simulink model "My_Model"  (R2022a)
settings: Solver=VariableStepAuto  StartTime=0.0  StopTime=10.0  RelTol=1e-3
libraries: neural x1294, spsSeriesRLCBranchLib x16, spsDiodeLib x14, spsMosfetLib x9, spsVoltageMeasurementLib x9, powerlib_extras x8, spsThreePhaseVIMeasurementLib x7, spsCurrentMeasurementLib x4, spsPVArrayLib x4, spsPWMGeneratorDCDCLib x4, spsTHDLib x4, spsThreePhaseParallelRLCBranchLib x3
(part 1 of 41)
settings Model: Creator=Irfan  LastModifiedBy=Irfan
settings SolverCC: MaxZcPerStep=1

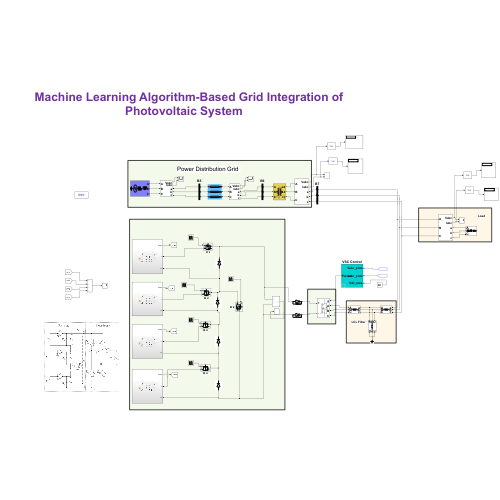
[thumbnail: Simulink's stored preview of the top-level diagram]
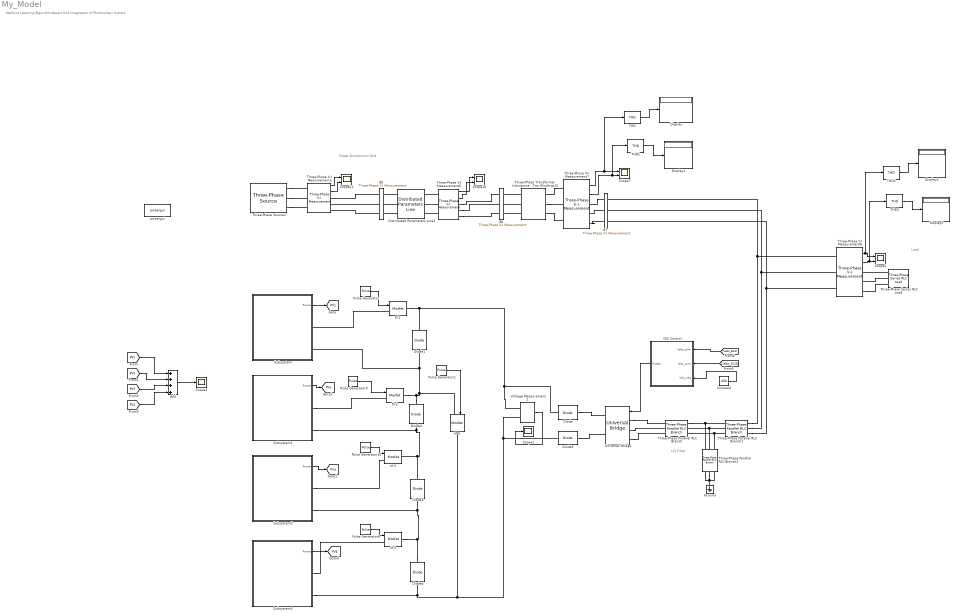
== system My_Model ==
  note: Load
  note: LCL Filter
  note: Machine Learning Algorithm-Based Grid Integration of Photovoltaic System
  note: Power Distribution Grid
  Add : Sum  Inputs=++++
  B5 : spsThreePhaseVIMeasurementLib/Three-Phase V-I Measurement  VoltageMeasurement=no  SetLabelV=off  LabelV=Vabc_B12  Vpu=off  VpuLL=off  CurrentMeasurement=no  SetLabelI=off  LabelI=A1  Ipu=off  Pbase=100e6  Vbase=25e3  OutputType=Magnitude  PhasorSimulation=off  PSBequivalent=0
  B6 : spsThreePhaseVIMeasurementLib/Three-Phase V-I Measurement  VoltageMeasurement=no  SetLabelV=off  LabelV=Vabc_B12  Vpu=off  VpuLL=off  CurrentMeasurement=no  SetLabelI=off  LabelI=A1  Ipu=off  Pbase=100e6  Vbase=440  OutputType=Magnitude  PhasorSimulation=off  PSBequivalent=0
  B7 : spsThreePhaseVIMeasurementLib/Three-Phase V-I Measurement  VoltageMeasurement=phase-to-ground  SetLabelV=on  LabelV=Vabc_B13  Vpu=off  VpuLL=off  CurrentMeasurement=yes  SetLabelI=on  LabelI=Iabc_b13  Ipu=off  Pbase=100e6  Vbase=440  OutputType=Magnitude  PhasorSimulation=off  PSBequivalent=0
  Constant : Constant  Value=400
  Diode : spsDiodeLib/Diode  Ron=0.001  Lon=0  Vf=0.8  IC=0  UseSnubber=0  Rs=500  Cs=250e-9  Measurements=off
  Diode{1..4} (4 alike) : spsDiodeLib/Diode  Ron=0.001  Lon=0  Vf=0.7  IC=0  UseSnubber=0  Rs=500  Cs=0  Measurements=off
  Diode5 : spsDiodeLib/Diode  Ron=0.001  Lon=0  Vf=0.8  IC=0  UseSnubber=0  Rs=500  Cs=250e-9  Measurements=off
  Display{,1..3} (4 alike) : Display
  Distributed Parameters Line1 : spsDistributedParametersLineLib/Distributed Parameters Line  Phases=3  Length=100  Frequency=50  Resistance=[0.01273 0.3864]  Inductance="[0.9337e-3  4.1264e-3]"  Capacitance=[12.74e-9 7.751e-9]  x1=[-0.0006 -0.058188576465129 21083.6440305902 -61014.2835927059;-0.00055 -0.0555200850052596 22039.4110790569 -60675.591993026;-0.0005 -0.0528378947951801 22989.7402326226 -60321.9295989302;-0.00045 -0.0501426676251903 23934.3970117888 -59953.3836713222;-0.0004 -0.0474350685022648 24873.1483366304 -59570.0451433951;-0.00035 -0.0447157654859725 25805.7625843049 -59172.0085981946;-0.0003 -0.0419854295236429 26732.0096462016 -58759.3722452823;-0.00025 -0.0392447342848198 27651.6609847177 -58332.2378965037;-0.0002 -0.0364943559950435 28564.4896896465 -57890.7109408683;-0.00015 -0.0337349732690022 29470.2705341641 -57434.9003185455;-0.0001 -0.0309672669430941 30368.7800304004 -56964.9184939859;-5e-05 -0.0281919199074408 31259.7964845821 -56480.8814281723]  x2=[-0.0006 -0.327906164256312 21190.0392255692 -61379.0148200665;-0.00055 -0.31698546988336 22151.5200142409 -61038.6090322539;-0.0005 -0.305986564088869 23107.5352468095 -60683.1428810029;-0.00045 -0.294912160688264 24057.8490408213 -60312.7040722674;-0.0004 -0.283764992124876 25002.2269205677 -59927.3840062804;-0.00035 -0.272547808795747 25940.4358749378 -59527.2777550025;-0.0003 -0.261263378373018 26872.2444149108 -59112.4840386644;-0.00025 -0.249914485121043 27797.4226306725 -58683.1052014089;-0.0002 -0.238503929209416 28715.7422483418 -58239.247186039;-0.00015 -0.227034526022067 29626.9766862941 -57781.0195078786;-0.0001 -0.215509105462612 30530.9011110672 -57308.5352277505;-5e-05 -0.203930511256117 31427.2924928347 -56821.910924081]  x3=[-0.0006 -0.00428228203564021 53.1676137199478 -232.949570816253;-0.00055 -0.0042908783266208 56.8201229832142 -232.085797433882;-0.0005 -0.00429841590758009 60.4586127313522 -231.164760353768;-0.00045 -0.00430489291873276 64.0821852214604 -230.186686828029;-0.0004 -0.00431030776197323 67.6899463912475 -229.151818181673;-0.00035 -0.00431465910126995 71.2810060796291 -228.060409753053;-0.0003 -0.00431794586299507 74.854478246361 -226.912730830867;-0.00025 -0.0043201672361893 78.4094811906572 -225.709064587717;-0.0002 -0.00432132267276205 81.9451377687359 -224.449708010237;-0.00015 -0.00432141188762664 85.4605756102416 -223.134971825819;-0.0001 -0.00432043485877063 88.9549273334895 -221.765180425943;-5e-05 -0.00431839182726127 92.4273307594791 -220.34067178614]  x4=[-0.0006 0.00367124666063104 77.9758993188108 -226.009964584727;-0.00055 0.00369703359433742 81.5162088738942 -224.757235875746;-0.0005 0.00372190834032431 85.0364055241912 -223.449051681928;-0.00045 0.00374586476112033 88.5356207138521 -222.085734778147;-0.0004 0.00376889694583712 92.0129910638889 -220.66762154245;-0.00035 0.00379099921162774 95.4676585852005 -219.195061873057;-0.0003 0.00381216610508883 98.8987708902695 -217.668419102034;-0.00025 0.00383239240360616 102.305481403475 -216.08806990564;-0.0002 0.00385167311664321 105.686949569975 -214.454404211391;-0.00015 0.00387000348697256 109.042341063096 -212.767825101854;-0.0001 0.0038873789918496 112.370827990194 -211.028748715186;-5e-05 0.0039037953441285 115.671589096928 -209.237604142463]  x5=0.000565541566995743  V1=[0 0 0 3.131e-09 6.455e+04 6.455e+04;0 0 0 314.2 314.2 314.2;1.571 1.571 1.571 -0.216 0.4129 -1.158]  V2=[0 0 0 1.333e-08 6.493e+04 6.493e+04;0 0 0 314.2 314.2 314.2;1.571 1.571 1.571 -0.3355 0.4126 -1.158]  I1=[0 0 0 7.522e-11 238.9 238.9;0 0 0 314.2 314.2 314.2;1.571 1.571 1.571 -1.605 0.3047 -1.266]  I2=[0 0 0 7.015e-11 239.1 239.1;0 0 0 314.2 314.2 314.2;1.571 1.571 1.571 1.244 0.4122 -1.159]  nHarmo=2  Measurements=None  Decoupling=off  VsMag0=0  VrMag0=0  VsAngle0=0  VrAngle0=0  IsMag0=0  IrMag0=0  IsAngle0=0  IrAngle0=0
      settings: SourceProductBaseCode=PS
  Ground : spsGroundLib/Ground  LConnTagsString=a
  M {1..4,9} (5 alike) : spsMosfetLib/Mosfet  Ron=0.1  Lon=0  Rd=0.01  Vfd=0  IC=0  Rs=1e5  Cs=inf  Measurements=off
  Pulse Generator : DiscretePulseGenerator  PulseType=Time based  Period=0.01  PulseWidth=99.999999
  Pulse Generator1 : DiscretePulseGenerator  PulseType=Time based  Amplitude=0  Period=0.01  PulseWidth=50  PhaseDelay=0.0026
  Pulse Generator10 : DiscretePulseGenerator  PulseType=Time based  Period=0.01  PulseWidth=50  PhaseDelay=0.0026
  Pulse Generator8 : DiscretePulseGenerator  PulseType=Time based  Period=0.01  PulseWidth=25  PhaseDelay=0.0039
  Pulse Generator9 : DiscretePulseGenerator  PulseType=Time based  Period=0.01  PulseWidth=75  PhaseDelay=0.0013
  Scope1 : Scope
  Scope{5,7,10..11} (4 alike) : Scope  NumInputPorts=2
  Scope2 : Scope
  Subsystem : Subsystem
  Subsystem1 : Subsystem
  Subsystem2 : Subsystem
  Subsystem3 : Subsystem
  THD{,1..3} (4 alike) : spsTHDLib/THD  Freq=60  Ts=0
      settings: SourceProductBaseCode=PS
  Three-Phase Parallel RLC Branch : spsThreePhaseParallelRLCBranchLib/Three-Phase Parallel RLC Branch  LConnTagsString=A|B|C  RConnTagsString=A|B|C  BranchType=L  Resistance=1  Inductance=2e-1  Capacitance=1e-6  Measurements=None
      settings: SourceProductBaseCode=PS
  Three-Phase Parallel RLC Branch1 : spsThreePhaseParallelRLCBranchLib/Three-Phase Parallel RLC Branch  LConnTagsString=A|B|C  RConnTagsString=A|B|C  BranchType=L  Resistance=1  Inductance=2e-1  Capacitance=1e-6  Measurements=None
      settings: SourceProductBaseCode=PS
  Three-Phase Parallel RLC Branch2 : spsThreePhaseParallelRLCBranchLib/Three-Phase Parallel RLC Branch  LConnTagsString=A|B|C  RConnTagsString=A|B|C  BranchType=C  Resistance=1  Inductance=1e-3  Capacitance=500e-5  Measurements=None
      settings: SourceProductBaseCode=PS
  Three-Phase Series RLC Load : spsThreePhaseSeriesRLCLoadLib/Three-Phase Series RLC Load  LConnTagsString=A|B|C  Configuration=Y (grounded)  NominalVoltage=440  Vabc=[440 440 440]  Vabcp=[1e3 1e3 1e3]  NominalFrequency=50  UnbalancedPower=on  ActivePower=10e3  InductivePower=1000  CapacitivePower=1000  Pabc=[10e3 9e3 11e3]  QLabc=[100 90 110]  QCabc=[100 90 110]  Pabcp=[10e3 9e3 11e3]  QLabcp=[100 90 110]  QCabcp=[100 90 110]  Measurements=None  LoadType=constant Z
  Three-Phase V-I Measurement5 : spsThreePhaseVIMeasurementLib/Three-Phase V-I Measurement  VoltageMeasurement=phase-to-ground  SetLabelV=off  LabelV=Vabc  Vpu=off  VpuLL=off  CurrentMeasurement=yes  SetLabelI=off  LabelI=Iabc  Ipu=off  Pbase=100e6  Vbase=500e3  OutputType=Complex  PhasorSimulation=off  PSBequivalent=0
  Three-Phase V-I Measurement6 : spsThreePhaseVIMeasurementLib/Three-Phase V-I Measurement  VoltageMeasurement=phase-to-ground  SetLabelV=off  LabelV=Vabc  Vpu=off  VpuLL=off  CurrentMeasurement=yes  SetLabelI=off  LabelI=Iabc  Ipu=off  Pbase=100e6  Vbase=500e3  OutputType=Complex  PhasorSimulation=off  PSBequivalent=0
  Three-Phase V-I Measurement7 : spsThreePhaseVIMeasurementLib/Three-Phase V-I Measurement  VoltageMeasurement=phase-to-phase  SetLabelV=off  LabelV=Vabc_b1  Vpu=off  VpuLL=off  CurrentMeasurement=yes  SetLabelI=off  LabelI=Iabc_b1  Ipu=off  Pbase=100e6  Vbase=500e3  OutputType=Complex  PhasorSimulation=off  PSBequivalent=0
  Three-Phase V-I Measurement8 : spsThreePhaseVIMeasurementLib/Three-Phase V-I Measurement  VoltageMeasurement=phase-to-phase  SetLabelV=off  LabelV=Vabc_b1  Vpu=off  VpuLL=off  CurrentMeasurement=yes  SetLabelI=off  LabelI=Iabc_b1  Ipu=off  Pbase=100e6  Vbase=500e3  OutputType=Complex  PhasorSimulation=off  PSBequivalent=0
  Three-Phase Source1 : spsThreePhaseSourceLib/Three-Phase Source  InternalConnection=Yg  VoltagePhases=off  Voltage=63510.4  PhaseAngle=0  Voltage_phases=[25e3 25e3 25e3]/sqrt(3)  PhaseAngles_phases=[0 -120 +120]  Frequency=50  NonIdealSource=on  SpecifyImpedance=on  Resistance=0.8929  Inductance=16.58e-3  ShortCircuitLevel=100e6  BaseVoltage=63510.4  XRratio=7  BusType=swing  Pref=0  Qref=0  Prefabc=[10e3, 10e3, 10e3]  Qrefabc=[0, 0, 0]  Qmin=-inf  Qmax=inf
  Three-Phase Transformer Inductance Matrix Type (Two Windings)3 : spsThreePhaseTransformerInductanceMatrixTypeTwoWindingsLib/Three-Phase Transformer Inductance Matrix Type (Two Windings)  CoreType=Three-limb or five-limb core  Winding1Connection=Yg  Winding2Connection=Yg  AutoTransformer=off  Measurements=None  NominalPower=[100e3 50]  VLLnom=[63510.4 254.03]  WindingResistances=[0.01 0.01]  NoLoadIexcPos=2  NoLoadPlossPos=1000  ShortCircuitReactancePos=0.06  ShortCircuitReactancePosAuto=0.06  NoLoadIexcZero=100  NoLoadPlossZero=1500  ShortCircuitReactanceZero=0.03  ShortCircuitReactanceZeroAuto=0.03
      settings: SourceProductBaseCode=PS
  Universal Bridge : spsUniversalBridgeLib/Universal Bridge  Arms=3  SnubberResistance=1e5  SnubberCapacitance=inf  Device=MOSFET / Diodes  Ron=1e-3  Lon=0  ForwardVoltages="[  0  0  ]"  ForwardVoltage=0  GTOparameters=[ 10e-6 , 20e-6 ]  IGBTparameters=[ 1e-6 , 2e-6 ]  Measurements=None  Measurements_2=None  converterType=Rectifier
  VSC Control : Subsystem  mask(VSC Main Controller){nom=[ 100e3  50 ], Vnom=[ 440 440 ], Vnom_dc=440, RLxfo=[0.002  0.06 ], RLchoke=[2e-3  250e-6  ], K_VDCreg=[7  800], K_Ireg=[0.3 20], Ts=50e-6}
      mask prompts: nom "Nominal power and frequency [ Pnom(VA)  Fnom(Hz) ]:"; Vnom "Nominal primary and secondary voltages (Vrms LL) [ Vnom_prim   Vnom_sec ]:"; Vnom_dc "Nominal DC bus voltage (V):"; RLxfo "Total transformer leakage impedance (pu/Pnom) [ Rxfo  Lxf ]"; RLchoke "Choke impedance [ R(ohm) L(H) ]"; K_VDCreg "VDC regultator gains [ Kp  Ki ]:"; K_Ireg "Current regulator gains [ Kp  Ki ]:"; Ts "Sample time"
      mask init:
      | Pnom=nom(1);
      | Fnom=nom(2);
      | Vnom_prim=Vnom(1);
      | Vnom_sec=Vnom(2);
      | Zbase=Vnom_sec^2/Pnom;
      | Rtot_pu=RLxfo(1) + RLchoke(1)/Zbase;
      | Ltot_pu=RLxfo(2) + RLchoke(2)/(Zbase/(2*pi*Fnom));
      | Kp_VDCreg=K_VDCreg(1);
      | Ki_VDCreg=K_VDCreg(2);
      | Kp_Ireg=K_Ireg(1);
      | Ki_Ireg=K_Ireg(2);
      | Vdc_ref=Vnom_dc;
      | % Used to determine initial value of Boost Control (MPPT)
      | assignin('base','Vdc_ref_Inv',Vdc_ref);
  Voltage Measurement1 : spsVoltageMeasurementLib/Voltage Measurement  PhasorSimulation=off  OutputType=Complex  PSBequivalent=0
  powergui : spspowerguiLib/powergui  Priority=1  SimulationMode=Discrete  SampleTime=50e-6  frequency=60  Iterations=50  frequencyindice=0  Pbase=100e6  ErrMax=1e-4  UnitsV=kV  UnitsW=MW  buscounter=0  FunctionMessages=off  echomessages=off  EnableUseOfTLC=off  CurrentSourceSwitches=off  DisableSnubberDevices=off  DisableRonSwitches=off  DisableVfSwitches=off  DisplayEquations=off  AutomaticDiscreteSolvers=off  SolverType=Tustin/Backward Euler (TBE)  Interpol=off  ExternalGateDelay=off  methode=off  Ts=100  x0status=blocks  SPID=on  SwTol=0  HookPort=off  NonlinearTolerance=1e-4  nMaxIteration=100  ContinueOnMaxIteration=off  RestoreLinks=warning  ResistiveCurrentMeasurement=off  Frange=[0:2:500]  Ylog=off  Xlog=on  ShowGrid=off  save=off  variable=ZData  structure=LD  ZoomFFT=off  StartTime=0.0  cycles=3  DisplayStyle=1  fundamental=50  FreqAxis=off  MaxFrequency=1000  frequencyindicesteady=1  RmsSteady=1  display=off
  tag scope: PV1=global, PV2=global, PV3=global, PV4=global
  wires:
  THD2/1 -> Display2/1
  Three-Phase V-I Measurement8/2 -> THD3/1, Scope5/2
  THD/1 -> Display/1
  Three-Phase V-I Measurement8/1 -> THD2/1, Scope5/1
  Subsystem3/1(Power) -> [PV4]
  Pulse Generator/1 -> M 1/1
  [PV4] -> Add/4
  Three-Phase V-I Measurement7/1 -> THD/1, Scope7/1
  Three-Phase V-I Measurement7/2 -> THD1/1, Scope7/2
  THD3/1 -> Display3/1
  Three-Phase V-I Measurement6/1 -> Scope10/1
  VSC Control/1(Pulses) -> Universal Bridge/1
  [Iabc_b13] -> VSC Control/2(Iabc_prim)
  [PV3] -> Add/3
  Constant/1 -> VSC Control/3(Vdc_mes)
  Three-Phase V-I Measurement5/2 -> Scope11/2
  [Vabc_B13] -> VSC Control/1(Vabc_prim)
  Pulse Generator1/1 -> M 9/1
  Subsystem1/1(Power) -> [PV2]
  Three-Phase V-I Measurement6/2 -> Scope10/2
  Subsystem/1(Power) -> [PV1]
  Add/1 -> Scope2/1
  Subsystem2/1(Power) -> [PV3]
  [PV2] -> Add/2
  Three-Phase V-I Measurement5/1 -> Scope11/1
  THD1/1 -> Display1/1
  [PV1] -> Add/1
  Voltage Measurement1/1 -> Scope1/1
  Pulse Generator10/1 -> M 3/1
  Pulse Generator8/1 -> M 4/1
  Pulse Generator9/1 -> M 2/1
  connections:
  Three-Phase Parallel RLC Branch2/LConn1 -- Three-Phase Parallel RLC Branch1/LConn1 -- Three-Phase Parallel RLC Branch/RConn1
  Diode/LConn1 -- Voltage Measurement1/LConn1 -- M 1/RConn1 -- Diode1/RConn1
  Three-Phase Parallel RLC Branch2/LConn3 -- Three-Phase Parallel RLC Branch/RConn3 -- Three-Phase Parallel RLC Branch1/LConn3
  M 9/RConn1 -- Subsystem3/RConn2 -- Diode4/LConn1 -- Diode5/LConn1 -- Voltage Measurement1/LConn2
  Diode2/RConn1 -- Diode1/LConn1 -- Subsystem/RConn2 -- M 9/LConn1 -- M 2/RConn1
  Three-Phase V-I Measurement8/LConn1 -- Three-Phase Parallel RLC Branch1/RConn1 -- B7/LConn1
  Three-Phase V-I Measurement8/LConn2 -- Three-Phase Parallel RLC Branch1/RConn2 -- B7/LConn2
  B7/LConn3 -- Three-Phase Parallel RLC Branch1/RConn3 -- Three-Phase V-I Measurement8/LConn3
  Diode4/RConn1 -- Subsystem2/RConn2 -- Diode3/LConn1 -- M 4/RConn1
  Three-Phase Parallel RLC Branch2/RConn2 -- Three-Phase Parallel RLC Branch2/RConn3 -- Three-Phase Parallel RLC Branch2/RConn1 -- Ground/LConn1
  Diode2/LConn1 -- Diode3/RConn1 -- M 3/RConn1 -- Subsystem1/RConn2
  Three-Phase Parallel RLC Branch2/LConn2 -- Three-Phase Parallel RLC Branch/RConn2 -- Three-Phase Parallel RLC Branch1/LConn2
  Three-Phase V-I Measurement8/RConn3 -- Three-Phase Series RLC Load/LConn3
  Subsystem3/RConn1 -- M 4/LConn1
  Three-Phase V-I Measurement6/RConn2 -- B6/RConn2
  Universal Bridge/LConn1 -- Three-Phase Parallel RLC Branch/LConn1
  Diode/RConn1 -- Universal Bridge/RConn1
  Three-Phase Transformer Inductance Matrix Type (Two Windings)3/LConn3 -- B6/LConn3
  Three-Phase V-I Measurement6/LConn3 -- Distributed Parameters Line1/RConn3
  Three-Phase Transformer Inductance Matrix Type (Two Windings)3/LConn2 -- B6/LConn2
  M 1/LConn1 -- Subsystem/RConn1
  Three-Phase Source1/RConn1 -- Three-Phase V-I Measurement5/LConn1
  B5/RConn1 -- Three-Phase V-I Measurement5/RConn1
  Three-Phase Series RLC Load/LConn2 -- Three-Phase V-I Measurement8/RConn2
  Three-Phase V-I Measurement6/RConn3 -- B6/RConn3
  B5/RConn2 -- Three-Phase V-I Measurement5/RConn2
  Distributed Parameters Line1/LConn1 -- B5/LConn1
  Three-Phase Source1/RConn3 -- Three-Phase V-I Measurement5/LConn3
  Three-Phase V-I Measurement6/LConn1 -- Distributed Parameters Line1/RConn1
  Three-Phase Transformer Inductance Matrix Type (Two Windings)3/RConn2 -- Three-Phase V-I Measurement7/LConn2
  B5/RConn3 -- Three-Phase V-I Measurement5/RConn3
  Subsystem1/RConn1 -- M 2/LConn1
  Distributed Parameters Line1/LConn3 -- B5/LConn3
  Three-Phase V-I Measurement7/RConn2 -- B7/RConn2
  Three-Phase Transformer Inductance Matrix Type (Two Windings)3/LConn1 -- B6/LConn1
  Three-Phase V-I Measurement7/RConn3 -- B7/RConn3
  Three-Phase Transformer Inductance Matrix Type (Two Windings)3/RConn1 -- Three-Phase V-I Measurement7/LConn1
  Subsystem2/RConn1 -- M 3/LConn1
  Three-Phase Series RLC Load/LConn1 -- Three-Phase V-I Measurement8/RConn1
  Distributed Parameters Line1/LConn2 -- B5/LConn2
  Universal Bridge/LConn3 -- Three-Phase Parallel RLC Branch/LConn3
  Three-Phase V-I Measurement6/LConn2 -- Distributed Parameters Line1/RConn2
  Universal Bridge/LConn2 -- Three-Phase Parallel RLC Branch/LConn2
  Three-Phase V-I Measurement7/RConn1 -- B7/RConn1
  Three-Phase Transformer Inductance Matrix Type (Two Windings)3/RConn3 -- Three-Phase V-I Measurement7/LConn3
  Diode5/RConn1 -- Universal Bridge/RConn2
  Three-Phase Source1/RConn2 -- Three-Phase V-I Measurement5/LConn2
  Three-Phase V-I Measurement6/RConn1 -- B6/RConn1

== system My_Model/Subsystem ==
  Constant : Constant  Value=1000
  Constant1 : Constant  Value=25
  Current Measurement1 : spsCurrentMeasurementLib/Current Measurement  PhasorSimulation=off  OutputType=Complex  PSBequivalent=0
  Custom Neural Network1 : Subsystem
      mask help: Custom Neural Network
      mask Display: e = 0.06;c1 = [120 150 230]/255;c2 = ([120 150 230]+0)/383;c3 = ([120 150 230]+128)/383;patch([0 1 1 0],[0 0 1 1],c1);patch([0 1 1 1-e 1-e 0+e],[0 0 1 1-e 0+e 0+e],c2);patch([0 0 1 1-e 0+e 0+e],[0 1 1 1-e 1-e 0+e],c3);plot([0 1 1 0 0],[0 0 1 1 0]);fprintf('NNET');port_label('input',1,' Input');port_label('output',1,'Output ');
  Demux : Demux  Outputs=5
  Diode : spsDiodeLib/Diode  Ron=0.5  Lon=0  Vf=0.7  IC=0  UseSnubber=0  Rs=1e5  Cs=250e-9  Measurements=off
  Diode1 : spsDiodeLib/Diode  Ron=0.5  Lon=0  Vf=0.7  IC=0  UseSnubber=0  Rs=1e5  Cs=250e-9  Measurements=off
  MPPT Power : Product
  Mosfet : spsMosfetLib/Mosfet  Ron=0.1  Lon=0  Rd=0.01  Vfd=0.7  IC=0  Rs=1e5  Cs=inf  Measurements=off
  Mux : Mux  Inputs=2
  Mux1 : Mux  Inputs=2
  PV Array : spsPVArrayLib/PV Array  Npar=5  Nser=10  PlotType=array @ 1000 W/m2 & specified temperatures  S_vec="[ 1000  500  100 ]"  Temp_C_vec="[ 45 25  ]"  ModuleName=User-defined  PlotWhenSelected=off  Pm=213.15  Ncell=60  Voc=36.3  Isc=7.84  Vm=29  Im=7.35  beta_Voc_pc=-0.36099  alpha_Isc_pc=0.102  beta_Voc=-0.13104  alpha_Isc=0.0079968  IL=7.8654  I0=2.9273e-10  nI=0.98119  Rsh=313.0553  Rs=0.39381  RobustModel=off  RobustCellTemperature=25  BAL=on  Tc=1e-6  Tfilter=5e-5
  PV Power : Product
  PWM Generator (DC-DC) : spsPWMGeneratorDCDCLib/PWM Generator (DC-DC)  Fsw=3000  Ts=0
  Scope : Scope  NumInputPorts=5
  Scope{1..3,5} (4 alike) : Scope
  Scope6 : Scope  NumInputPorts=3
  Scope7 : Scope  NumInputPorts=3
  Series RLC Branch : spsSeriesRLCBranchLib/Series RLC Branch  LConnTagsString=__new0  RConnTagsString=__new0  BranchType=L  Resistance=0.001  Inductance=0.4e-1  SetiL0=off  InitialCurrent=0  Capacitance=1e-6  Setx0=off  InitialVoltage=0  Measurements=None
  Series RLC Branch1 : spsSeriesRLCBranchLib/Series RLC Branch  LConnTagsString=__new0  RConnTagsString=__new0  BranchType=R  Resistance=18  Inductance=0.1  SetiL0=off  InitialCurrent=0  Capacitance=100e-6  Setx0=off  InitialVoltage=0  Measurements=None
  Series RLC Branch2 : spsSeriesRLCBranchLib/Series RLC Branch  LConnTagsString=__new0  RConnTagsString=__new0  BranchType=C  Resistance=6  Inductance=0.1  SetiL0=off  InitialCurrent=0  Capacitance=700e-5  Setx0=off  InitialVoltage=0  Measurements=None
  Series RLC Branch3 : spsSeriesRLCBranchLib/Series RLC Branch  LConnTagsString=__new0  RConnTagsString=__new0  BranchType=C  Resistance=6  Inductance=0.1  SetiL0=off  InitialCurrent=0  Capacitance=900e-5  Setx0=off  InitialVoltage=0  Measurements=None
  Temp2 : powerlib_extras/Control  Blocks/Timer  t=[0 .1 .2 .3 .4 .5 .6 .7 .8 .9 1 ]  e=[20 23 25 25 26 27 28 25 24 25 25]
      settings: SourceProductBaseCode=PS
  Voltage Measurement : spsVoltageMeasurementLib/Voltage Measurement  PhasorSimulation=off  OutputType=Complex  PSBequivalent=0
  Voltage Measurement1 : spsVoltageMeasurementLib/Voltage Measurement  PhasorSimulation=off  OutputType=Complex  PSBequivalent=0
  irr 2 : powerlib_extras/Control  Blocks/Timer  t=[0 0.05 0.1 .15 .2 .25 .3 .35 0.4 .45 .5 .6 .7 .8 0.9 1 ]  e=[250 500 500 500 600 700 800 1000 1000 1000 1000 1000 1000 1000 1000 1000]
      settings: SourceProductBaseCode=PS
  k : PMIOPort  Side=Right
  k1 : PMIOPort  Port=2  Side=Right
  Power : Outport  VectorParamsAs1DForOutWhenUnconnected=off
  wires:
  Constant1/1 -> PV Array/2
  Demux/1 -> Scope/1, Mux/1, PV Power/1, Scope7/1  "PV Voltage"
  Mux/1 -> Custom Neural Network1/1(Input)
  MPPT Power/1 -> Scope2/1, Power/1, Scope6/2  "CNFF"
  Demux/2 -> Scope/2, Mux/2, PV Power/2
  Custom Neural Network1/1(Output) -> PWM Generator (DC-DC)/1
  Current Measurement1/1 -> Mux1/1, MPPT Power/1
  PV Array/1 -> Demux/1
  Voltage Measurement/1 -> Scope7/2, Mux1/2, MPPT Power/2  "DC -DC Boost Converter Voltage"
  Demux/5 -> Scope/5
  Constant/1 -> PV Array/1
  PWM Generator (DC-DC)/1 -> Mosfet/1
  Mux1/1 -> Scope1/1
  PV Power/1 -> Scope5/1, Scope6/1
  Voltage Measurement1/1 -> Scope3/1
  Demux/4 -> Scope/4, Scope7/3, Scope6/3  "Irradiance"
  Demux/3 -> Scope/3
  connections:
  Series RLC Branch/LConn1 -- Diode1/RConn1 -- PV Array/RConn1 -- Series RLC Branch2/LConn1
  Current Measurement1/LConn1 -- Diode/RConn1 -- Series RLC Branch3/LConn1
  Diode/LConn1 -- Mosfet/LConn1 -- Series RLC Branch/RConn1 -- Voltage Measurement1/LConn1
  Current Measurement1/RConn1 -- Series RLC Branch1/LConn1 -- k/RConn1 -- Voltage Measurement/LConn1
  Diode1/LConn1 -- PV Array/RConn2 -- Series RLC Branch2/RConn1 -- Mosfet/RConn1 -- Voltage Measurement1/LConn2 -- Series RLC Branch3/RConn1 -- Series RLC Branch1/RConn1 -- k1/RConn1 -- Voltage Measurement/LConn2

== system My_Model/Subsystem1 ==
  Constant : Constant  Value=1000
  Constant1 : Constant  Value=25
  Current Measurement1 : spsCurrentMeasurementLib/Current Measurement  PhasorSimulation=off  OutputType=Complex  PSBequivalent=0
  Custom Neural Network1 : Subsystem
      mask help: Custom Neural Network
      mask Display: e = 0.06;c1 = [120 150 230]/255;c2 = ([120 150 230]+0)/383;c3 = ([120 150 230]+128)/383;patch([0 1 1 0],[0 0 1 1],c1);patch([0 1 1 1-e 1-e 0+e],[0 0 1 1-e 0+e 0+e],c2);patch([0 0 1 1-e 0+e 0+e],[0 1 1 1-e 1-e 0+e],c3);plot([0 1 1 0 0],[0 0 1 1 0]);fprintf('NNET');port_label('input',1,' Input');port_label('output',1,'Output ');
  Demux : Demux  Outputs=5
  Diode : spsDiodeLib/Diode  Ron=0.5  Lon=0  Vf=0.7  IC=0  UseSnubber=0  Rs=1e5  Cs=250e-9  Measurements=off
  Diode1 : spsDiodeLib/Diode  Ron=0.5  Lon=0  Vf=0.7  IC=0  UseSnubber=0  Rs=1e5  Cs=250e-9  Measurements=off
  MPPT Power : Product
  Mosfet : spsMosfetLib/Mosfet  Ron=0.1  Lon=0  Rd=0.01  Vfd=0.7  IC=0  Rs=1e5  Cs=inf  Measurements=off
  Mux : Mux  Inputs=2
  Mux1 : Mux  Inputs=2
  PV Array : spsPVArrayLib/PV Array  Npar=5  Nser=10  PlotType=array @ 1000 W/m2 & specified temperatures  S_vec="[ 1000  500  100 ]"  Temp_C_vec="[ 45 25  ]"  ModuleName=User-defined  PlotWhenSelected=off  Pm=213.15  Ncell=60  Voc=36.3  Isc=7.84  Vm=29  Im=7.35  beta_Voc_pc=-0.36099  alpha_Isc_pc=0.102  beta_Voc=-0.13104  alpha_Isc=0.0079968  IL=7.8654  I0=2.9273e-10  nI=0.98119  Rsh=313.0553  Rs=0.39381  RobustModel=off  RobustCellTemperature=25  BAL=on  Tc=1e-6  Tfilter=5e-5
  PV Power : Product
  PWM Generator (DC-DC) : spsPWMGeneratorDCDCLib/PWM Generator (DC-DC)  Fsw=3000  Ts=0
  Scope : Scope  NumInputPorts=5
  Scope{1..3,5} (4 alike) : Scope
  Scope6 : Scope  NumInputPorts=3
  Scope7 : Scope  NumInputPorts=3
  Series RLC Branch : spsSeriesRLCBranchLib/Series RLC Branch  LConnTagsString=__new0  RConnTagsString=__new0  BranchType=L  Resistance=0.001  Inductance=0.4e-1  SetiL0=off  InitialCurrent=0  Capacitance=1e-6  Setx0=off  InitialVoltage=0  Measurements=None
  Series RLC Branch1 : spsSeriesRLCBranchLib/Series RLC Branch  LConnTagsString=__new0  RConnTagsString=__new0  BranchType=R  Resistance=18  Inductance=0.1  SetiL0=off  InitialCurrent=0  Capacitance=100e-6  Setx0=off  InitialVoltage=0  Measurements=None
  Series RLC Branch2 : spsSeriesRLCBranchLib/Series RLC Branch  LConnTagsString=__new0  RConnTagsString=__new0  BranchType=C  Resistance=6  Inductance=0.1  SetiL0=off  InitialCurrent=0  Capacitance=700e-5  Setx0=off  InitialVoltage=0  Measurements=None
  Series RLC Branch3 : spsSeriesRLCBranchLib/Series RLC Branch  LConnTagsString=__new0  RConnTagsString=__new0  BranchType=C  Resistance=6  Inductance=0.1  SetiL0=off  InitialCurrent=0  Capacitance=900e-5  Setx0=off  InitialVoltage=0  Measurements=None
  Temp2 : powerlib_extras/Control  Blocks/Timer  t=[0 .1 .2 .3 .4 .5 .6 .7 .8 .9 1 ]  e=[20 23 25 25 26 27 28 25 24 25 25]
      settings: SourceProductBaseCode=PS
  Voltage Measurement : spsVoltageMeasurementLib/Voltage Measurement  PhasorSimulation=off  OutputType=Complex  PSBequivalent=0
  Voltage Measurement1 : spsVoltageMeasurementLib/Voltage Measurement  PhasorSimulation=off  OutputType=Complex  PSBequivalent=0
  irr 2 : powerlib_extras/Control  Blocks/Timer  t=[0 0.05 0.1 .15 .2 .25 .3 .35 0.4 .45 .5 .6 .7 .8 0.9 1 ]  e=[250 500 500 500 600 700 800 1000 1000 1000 1000 1000 1000 1000 1000 1000]
      settings: SourceProductBaseCode=PS
  k : PMIOPort  Side=Right
  k1 : PMIOPort  Port=2  Side=Right
  Power : Outport  VectorParamsAs1DForOutWhenUnconnected=off
  wires:
  Demux/3 -> Scope/3
  Demux/4 -> Scope6/3, Scope7/3, Scope/4  "Irradiance"
  Voltage Measurement1/1 -> Scope3/1
  PV Power/1 -> Scope6/1, Scope5/1
  Mux1/1 -> Scope1/1
  PWM Generator (DC-DC)/1 -> Mosfet/1
  Constant/1 -> PV Array/1
  Demux/5 -> Scope/5
  Voltage Measurement/1 -> MPPT Power/2, Mux1/2, Scope7/2  "DC -DC Boost Converter Voltage"
  PV Array/1 -> Demux/1
  Current Measurement1/1 -> MPPT Power/1, Mux1/1
  Custom Neural Network1/1(Output) -> PWM Generator (DC-DC)/1
  Demux/2 -> PV Power/2, Mux/2, Scope/2
  MPPT Power/1 -> Scope6/2, Power/1, Scope2/1  "CNFF"
  Mux/1 -> Custom Neural Network1/1(Input)
  Demux/1 -> Scope7/1, PV Power/1, Mux/1, Scope/1  "PV Voltage"
  Constant1/1 -> PV Array/2
  connections:
  k1/RConn1 -- Voltage Measurement/LConn2 -- Series RLC Branch1/RConn1 -- Series RLC Branch3/RConn1 -- Voltage Measurement1/LConn2 -- Mosfet/RConn1 -- Series RLC Branch2/RConn1 -- PV Array/RConn2 -- Diode1/LConn1
  k/RConn1 -- Voltage Measurement/LConn1 -- Series RLC Branch1/LConn1 -- Current Measurement1/RConn1
  Voltage Measurement1/LConn1 -- Series RLC Branch/RConn1 -- Mosfet/LConn1 -- Diode/LConn1
  Series RLC Branch3/LConn1 -- Diode/RConn1 -- Current Measurement1/LConn1
  Series RLC Branch2/LConn1 -- PV Array/RConn1 -- Diode1/RConn1 -- Series RLC Branch/LConn1

== system My_Model/Subsystem2 ==
  Constant : Constant  Value=1000
  Constant1 : Constant  Value=25
  Current Measurement1 : spsCurrentMeasurementLib/Current Measurement  PhasorSimulation=off  OutputType=Complex  PSBequivalent=0
  Custom Neural Network1 : Subsystem
      mask help: Custom Neural Network
      mask Display: e = 0.06;c1 = [120 150 230]/255;c2 = ([120 150 230]+0)/383;c3 = ([120 150 230]+128)/383;patch([0 1 1 0],[0 0 1 1],c1);patch([0 1 1 1-e 1-e 0+e],[0 0 1 1-e 0+e 0+e],c2);patch([0 0 1 1-e 0+e 0+e],[0 1 1 1-e 1-e 0+e],c3);plot([0 1 1 0 0],[0 0 1 1 0]);fprintf('NNET');port_label('input',1,' Input');port_label('output',1,'Output ');
  Demux : Demux  Outputs=5
  Diode : spsDiodeLib/Diode  Ron=0.5  Lon=0  Vf=0.7  IC=0  UseSnubber=0  Rs=1e5  Cs=250e-9  Measurements=off
  Diode1 : spsDiodeLib/Diode  Ron=0.5  Lon=0  Vf=0.7  IC=0  UseSnubber=0  Rs=1e5  Cs=250e-9  Measurements=off
  MPPT Power : Product
  Mosfet : spsMosfetLib/Mosfet  Ron=0.1  Lon=0  Rd=0.01  Vfd=0.7  IC=0  Rs=1e5  Cs=inf  Measurements=off
  Mux : Mux  Inputs=2
  Mux1 : Mux  Inputs=2
  PV Array : spsPVArrayLib/PV Array  Npar=5  Nser=10  PlotType=array @ 1000 W/m2 & specified temperatures  S_vec="[ 1000  500  100 ]"  Temp_C_vec="[ 45 25  ]"  ModuleName=User-defined  PlotWhenSelected=off  Pm=213.15  Ncell=60  Voc=36.3  Isc=7.84  Vm=29  Im=7.35  beta_Voc_pc=-0.36099  alpha_Isc_pc=0.102  beta_Voc=-0.13104  alpha_Isc=0.0079968  IL=7.8654  I0=2.9273e-10  nI=0.98119  Rsh=313.0553  Rs=0.39381  RobustModel=off  RobustCellTemperature=25  BAL=on  Tc=1e-6  Tfilter=5e-5
  PV Power : Product
  PWM Generator (DC-DC) : spsPWMGeneratorDCDCLib/PWM Generator (DC-DC)  Fsw=3000  Ts=0
  Scope : Scope  NumInputPorts=5
  Scope{1..3,5} (4 alike) : Scope
  Scope6 : Scope  NumInputPorts=3
  Scope7 : Scope  NumInputPorts=3
  Series RLC Branch : spsSeriesRLCBranchLib/Series RLC Branch  LConnTagsString=__new0  RConnTagsString=__new0  BranchType=L  Resistance=0.001  Inductance=0.4e-1  SetiL0=off  InitialCurrent=0  Capacitance=1e-6  Setx0=off  InitialVoltage=0  Measurements=None
  Series RLC Branch1 : spsSeriesRLCBranchLib/Series RLC Branch  LConnTagsString=__new0  RConnTagsString=__new0  BranchType=R  Resistance=18  Inductance=0.1  SetiL0=off  InitialCurrent=0  Capacitance=100e-6  Setx0=off  InitialVoltage=0  Measurements=None
  Series RLC Branch2 : spsSeriesRLCBranchLib/Series RLC Branch  LConnTagsString=__new0  RConnTagsString=__new0  BranchType=C  Resistance=6  Inductance=0.1  SetiL0=off  InitialCurrent=0  Capacitance=700e-5  Setx0=off  InitialVoltage=0  Measurements=None
  Series RLC Branch3 : spsSeriesRLCBranchLib/Series RLC Branch  LConnTagsString=__new0  RConnTagsString=__new0  BranchType=C  Resistance=6  Inductance=0.1  SetiL0=off  InitialCurrent=0  Capacitance=900e-5  Setx0=off  InitialVoltage=0  Measurements=None
  Temp2 : powerlib_extras/Control  Blocks/Timer  t=[0 .1 .2 .3 .4 .5 .6 .7 .8 .9 1 ]  e=[20 23 25 25 26 27 28 25 24 25 25]
      settings: SourceProductBaseCode=PS
  Voltage Measurement : spsVoltageMeasurementLib/Voltage Measurement  PhasorSimulation=off  OutputType=Complex  PSBequivalent=0
  Voltage Measurement1 : spsVoltageMeasurementLib/Voltage Measurement  PhasorSimulation=off  OutputType=Complex  PSBequivalent=0
  irr 2 : powerlib_extras/Control  Blocks/Timer  t=[0 0.05 0.1 .15 .2 .25 .3 .35 0.4 .45 .5 .6 .7 .8 0.9 1 ]  e=[250 500 500 500 600 700 800 1000 1000 1000 1000 1000 1000 1000 1000 1000]
      settings: SourceProductBaseCode=PS
  k : PMIOPort  Side=Right
  k1 : PMIOPort  Port=2  Side=Right
  Power : Outport  VectorParamsAs1DForOutWhenUnconnected=off
  wires:
  Constant1/1 -> PV Array/2
  Demux/1 -> Scope/1, Mux/1, PV Power/1, Scope7/1  "PV Voltage"
  Mux/1 -> Custom Neural Network1/1(Input)
  MPPT Power/1 -> Scope2/1, Power/1, Scope6/2  "CNFF"
  Demux/2 -> Scope/2, Mux/2, PV Power/2
  Custom Neural Network1/1(Output) -> PWM Generator (DC-DC)/1
  Current Measurement1/1 -> Mux1/1, MPPT Power/1
  PV Array/1 -> Demux/1
  Voltage Measurement/1 -> Scope7/2, Mux1/2, MPPT Power/2  "DC -DC Boost Converter Voltage"
  Demux/5 -> Scope/5
  Constant/1 -> PV Array/1
  PWM Generator (DC-DC)/1 -> Mosfet/1
  Mux1/1 -> Scope1/1
  PV Power/1 -> Scope5/1, Scope6/1
  Voltage Measurement1/1 -> Scope3/1
  Demux/4 -> Scope/4, Scope7/3, Scope6/3  "Irradiance"
  Demux/3 -> Scope/3
  connections:
  Series RLC Branch/LConn1 -- Diode1/RConn1 -- PV Array/RConn1 -- Series RLC Branch2/LConn1
  Current Measurement1/LConn1 -- Diode/RConn1 -- Series RLC Branch3/LConn1
  Diode/LConn1 -- Mosfet/LConn1 -- Series RLC Branch/RConn1 -- Voltage Measurement1/LConn1
  Current Measurement1/RConn1 -- Series RLC Branch1/LConn1 -- Voltage Measurement/LConn1 -- k/RConn1
  Diode1/LConn1 -- PV Array/RConn2 -- Series RLC Branch2/RConn1 -- Mosfet/RConn1 -- Voltage Measurement1/LConn2 -- Series RLC Branch3/RConn1 -- Series RLC Branch1/RConn1 -- Voltage Measurement/LConn2 -- k1/RConn1

== system My_Model/Subsystem3 ==
  Constant : Constant  Value=1000
  Constant1 : Constant  Value=25
  Current Measurement1 : spsCurrentMeasurementLib/Current Measurement  PhasorSimulation=off  OutputType=Complex  PSBequivalent=0
  Custom Neural Network1 : Subsystem
      mask help: Custom Neural Network
      mask Display: e = 0.06;c1 = [120 150 230]/255;c2 = ([120 150 230]+0)/383;c3 = ([120 150 230]+128)/383;patch([0 1 1 0],[0 0 1 1],c1);patch([0 1 1 1-e 1-e 0+e],[0 0 1 1-e 0+e 0+e],c2);patch([0 0 1 1-e 0+e 0+e],[0 1 1 1-e 1-e 0+e],c3);plot([0 1 1 0 0],[0 0 1 1 0]);fprintf('NNET');port_label('input',1,' Input');port_label('output',1,'Output ');
  Demux : Demux  Outputs=5
  Diode : spsDiodeLib/Diode  Ron=0.5  Lon=0  Vf=0.7  IC=0  UseSnubber=0  Rs=1e5  Cs=250e-9  Measurements=off
  Diode1 : spsDiodeLib/Diode  Ron=0.5  Lon=0  Vf=0.7  IC=0  UseSnubber=0  Rs=1e5  Cs=250e-9  Measurements=off
  MPPT Power : Product
  Mosfet : spsMosfetLib/Mosfet  Ron=0.1  Lon=0  Rd=0.01  Vfd=0.7  IC=0  Rs=1e5  Cs=inf  Measurements=off
  Mux : Mux  Inputs=2
  Mux1 : Mux  Inputs=2
  PV Array : spsPVArrayLib/PV Array  Npar=5  Nser=10  PlotType=array @ 1000 W/m2 & specified temperatures  S_vec="[ 1000  500  100 ]"  Temp_C_vec="[ 45 25  ]"  ModuleName=User-defined  PlotWhenSelected=off  Pm=213.15  Ncell=60  Voc=36.3  Isc=7.84  Vm=29  Im=7.35  beta_Voc_pc=-0.36099  alpha_Isc_pc=0.102  beta_Voc=-0.13104  alpha_Isc=0.0079968  IL=7.8654  I0=2.9273e-10  nI=0.98119  Rsh=313.0553  Rs=0.39381  RobustModel=off  RobustCellTemperature=25  BAL=on  Tc=1e-6  Tfilter=5e-5
  PV Power : Product
  PWM Generator (DC-DC) : spsPWMGeneratorDCDCLib/PWM Generator (DC-DC)  Fsw=3000  Ts=0
  Scope : Scope  NumInputPorts=5
  Scope{1..3,5} (4 alike) : Scope
  Scope6 : Scope  NumInputPorts=3
  Scope7 : Scope  NumInputPorts=3
  Series RLC Branch : spsSeriesRLCBranchLib/Series RLC Branch  LConnTagsString=__new0  RConnTagsString=__new0  BranchType=L  Resistance=0.001  Inductance=0.4e-1  SetiL0=off  InitialCurrent=0  Capacitance=1e-6  Setx0=off  InitialVoltage=0  Measurements=None
  Series RLC Branch1 : spsSeriesRLCBranchLib/Series RLC Branch  LConnTagsString=__new0  RConnTagsString=__new0  BranchType=R  Resistance=18  Inductance=0.1  SetiL0=off  InitialCurrent=0  Capacitance=100e-6  Setx0=off  InitialVoltage=0  Measurements=None
  Series RLC Branch2 : spsSeriesRLCBranchLib/Series RLC Branch  LConnTagsString=__new0  RConnTagsString=__new0  BranchType=C  Resistance=6  Inductance=0.1  SetiL0=off  InitialCurrent=0  Capacitance=700e-5  Setx0=off  InitialVoltage=0  Measurements=None
  Series RLC Branch3 : spsSeriesRLCBranchLib/Series RLC Branch  LConnTagsString=__new0  RConnTagsString=__new0  BranchType=C  Resistance=6  Inductance=0.1  SetiL0=off  InitialCurrent=0  Capacitance=900e-5  Setx0=off  InitialVoltage=0  Measurements=None
  Temp2 : powerlib_extras/Control  Blocks/Timer  t=[0 .1 .2 .3 .4 .5 .6 .7 .8 .9 1 ]  e=[20 23 25 25 26 27 28 25 24 25 25]
      settings: SourceProductBaseCode=PS
  Voltage Measurement : spsVoltageMeasurementLib/Voltage Measurement  PhasorSimulation=off  OutputType=Complex  PSBequivalent=0
  Voltage Measurement1 : spsVoltageMeasurementLib/Voltage Measurement  PhasorSimulation=off  OutputType=Complex  PSBequivalent=0
  irr 2 : powerlib_extras/Control  Blocks/Timer  t=[0 0.05 0.1 .15 .2 .25 .3 .35 0.4 .45 .5 .6 .7 .8 0.9 1 ]  e=[250 500 500 500 600 700 800 1000 1000 1000 1000 1000 1000 1000 1000 1000]
      settings: SourceProductBaseCode=PS
  k : PMIOPort  Side=Right
  k1 : PMIOPort  Port=2  Side=Right
  Power : Outport  VectorParamsAs1DForOutWhenUnconnected=off
  wires:
  Demux/3 -> Scope/3
  Demux/4 -> Scope6/3, Scope7/3, Scope/4  "Irradiance"
  Voltage Measurement1/1 -> Scope3/1
  PV Power/1 -> Scope6/1, Scope5/1
  Mux1/1 -> Scope1/1
  PWM Generator (DC-DC)/1 -> Mosfet/1
  Constant/1 -> PV Array/1
  Demux/5 -> Scope/5
  Voltage Measurement/1 -> MPPT Power/2, Mux1/2, Scope7/2  "DC -DC Boost Converter Voltage"
  PV Array/1 -> Demux/1
  Current Measurement1/1 -> MPPT Power/1, Mux1/1
  Custom Neural Network1/1(Output) -> PWM Generator (DC-DC)/1
  Demux/2 -> PV Power/2, Mux/2, Scope/2
  MPPT Power/1 -> Scope6/2, Power/1, Scope2/1  "CNFF"
  Mux/1 -> Custom Neural Network1/1(Input)
  Demux/1 -> Scope7/1, PV Power/1, Mux/1, Scope/1  "PV Voltage"
  Constant1/1 -> PV Array/2
  connections:
  k1/RConn1 -- Voltage Measurement/LConn2 -- Series RLC Branch1/RConn1 -- Series RLC Branch3/RConn1 -- Voltage Measurement1/LConn2 -- Mosfet/RConn1 -- Series RLC Branch2/RConn1 -- PV Array/RConn2 -- Diode1/LConn1
  k/RConn1 -- Voltage Measurement/LConn1 -- Series RLC Branch1/LConn1 -- Current Measurement1/RConn1
  Voltage Measurement1/LConn1 -- Series RLC Branch/RConn1 -- Mosfet/LConn1 -- Diode/LConn1
  Series RLC Branch3/LConn1 -- Diode/RConn1 -- Current Measurement1/LConn1
  Series RLC Branch2/LConn1 -- PV Array/RConn1 -- Diode1/RConn1 -- Series RLC Branch/LConn1

== system My_Model/VSC Control ==
  note: VSC Main Controller
  Vabc_prim : Inport  PortDimensions=3
  Iabc_prim : Inport  Port=2  PortDimensions=3
  Vdc_mes : Inport  Port=3  PortDimensions=1
  Current Regulator : Subsystem
  Iq_ref : Constant  Value=0
  Mux : Mux  Inputs=2
  PLL & Measurements : Subsystem
  PWM Generator (2-Level) : spsPWMGenerator2LevelLib/PWM Generator (2-Level)  ModulatorType=Three-phase bridge (6 pulses)  ModulatorMode=Unsynchronized  Fc=2000  Pc=90  nF=27  MinMax="[ -1  1 ]"  SamplingTechnique=Natural  ModulatingSignals=off  m=0.8  Freq=60  Phase=0  Ts=0  ShowCarrierOutport=off
  Uabc_ref Generation max (m) = 1 : Subsystem
  Unit Delay : UnitDelay  SampleTime=50e-6  HasFrameUpgradeWarning=on
  VDC Regulator : Subsystem
  Vdc_ref1 : Constant  Value=Vdc_ref
  Pulses : Outport  VectorParamsAs1DForOutWhenUnconnected=off
  wires:
  VDC Regulator/1(Id_ref) -> Mux/1
  PLL & Measurements/1(wt) -> Uabc_ref Generation max (m) = 1/1(wt)
  Current Regulator/1(VdVq_conv) -> Uabc_ref Generation max (m) = 1/2(VdVq_conv)
  Iq_ref/1 -> Mux/2
  Mux/1 -> Current Regulator/3(IdIq_ref)
  PLL & Measurements/3(IdIq_prim) -> Current Regulator/2(IdIq_mes)
  PLL & Measurements/2(VdVq_prim) -> Current Regulator/1(VdVq_mes)
  Vdc_mes/1 -> VDC Regulator/1(Vdc_mes)
  Vabc_prim/1 -> PLL & Measurements/1(Vabc_prim)
  Iabc_prim/1 -> PLL & Measurements/2(Iabc_prim)
  Unit Delay/1 -> PWM Generator (2-Level)/1
  PWM Generator (2-Level)/1 -> Pulses/1
  Uabc_ref Generation max (m) = 1/1(Uabc_ref) -> Unit Delay/1
  Vdc_ref1/1 -> VDC Regulator/2(Vdc_ref)

== system My_Model/Subsystem/Custom Neural Network1 ==
  Input : Inport  PortDimensions=2
      mask Display: e = 0.06;c1 = [120 230 180]/255;c2 = ([120 230 180]+0)/(256+128);c3 = ([120 230 180]+128)/(256+128);patch([0 1 1 0],[0 0 1 1],c1);patch([0 1 1 1-e 1-e 0+e],[0 0 1 1-e 0+e 0+e],c2);patch([0 0 1 1-e 0+e 0+e],[0 1 1 1-e 1-e 0+e],c3);plot([0 1 1 0 0],[0 0 1 1 0]);
  Layer 1 : Subsystem
      mask Display: e = 0.06;c1 = [120 150 230]/255;c2 = ([120 150 230]+0)/383;c3 = ([120 150 230]+128)/383;patch([0 1 1 0],[0 0 1 1],c1);patch([0 1 1 1-e 1-e 0+e],[0 0 1 1-e 0+e 0+e],c2);patch([0 0 1 1-e 0+e 0+e],[0 1 1 1-e 1-e 0+e],c3);plot([0 1 1 0 0],[0 0 1 1 0]);
  Layer 2 : Subsystem
      mask Display: e = 0.06;c1 = [120 150 230]/255;c2 = ([120 150 230]+0)/383;c3 = ([120 150 230]+128)/383;patch([0 1 1 0],[0 0 1 1],c1);patch([0 1 1 1-e 1-e 0+e],[0 0 1 1-e 0+e 0+e],c2);patch([0 0 1 1-e 0+e 0+e],[0 1 1 1-e 1-e 0+e],c3);plot([0 1 1 0 0],[0 0 1 1 0]);
  Layer 3 : Subsystem
      mask Display: e = 0.06;c1 = [120 150 230]/255;c2 = ([120 150 230]+0)/383;c3 = ([120 150 230]+128)/383;patch([0 1 1 0],[0 0 1 1],c1);patch([0 1 1 1-e 1-e 0+e],[0 0 1 1-e 0+e 0+e],c2);patch([0 0 1 1-e 0+e 0+e],[0 1 1 1-e 1-e 0+e],c3);plot([0 1 1 0 0],[0 0 1 1 0]);
  Layer 4 : Subsystem
      mask Display: e = 0.06;c1 = [120 150 230]/255;c2 = ([120 150 230]+0)/383;c3 = ([120 150 230]+128)/383;patch([0 1 1 0],[0 0 1 1],c1);patch([0 1 1 1-e 1-e 0+e],[0 0 1 1-e 0+e 0+e],c2);patch([0 0 1 1-e 0+e 0+e],[0 1 1 1-e 1-e 0+e],c3);plot([0 1 1 0 0],[0 0 1 1 0]);
  Layer 5 : Subsystem
      mask Display: e = 0.06;c1 = [120 150 230]/255;c2 = ([120 150 230]+0)/383;c3 = ([120 150 230]+128)/383;patch([0 1 1 0],[0 0 1 1],c1);patch([0 1 1 1-e 1-e 0+e],[0 0 1 1-e 0+e 0+e],c2);patch([0 0 1 1-e 0+e 0+e],[0 1 1 1-e 1-e 0+e],c3);plot([0 1 1 0 0],[0 0 1 1 0]);
  Layer 6 : Subsystem
      mask Display: e = 0.06;c1 = [120 150 230]/255;c2 = ([120 150 230]+0)/383;c3 = ([120 150 230]+128)/383;patch([0 1 1 0],[0 0 1 1],c1);patch([0 1 1 1-e 1-e 0+e],[0 0 1 1-e 0+e 0+e],c2);patch([0 0 1 1-e 0+e 0+e],[0 1 1 1-e 1-e 0+e],c3);plot([0 1 1 0 0],[0 0 1 1 0]);
  Process Output 1 : Subsystem
      mask Display: e = 0.06;c1 = [120 150 230]/255;c2 = ([120 150 230]+0)/383;c3 = ([120 150 230]+128)/383;patch([0 1 1 0],[0 0 1 1],c1);patch([0 1 1 1-e 1-e 0+e],[0 0 1 1-e 0+e 0+e],c2);patch([0 0 1 1-e 0+e 0+e],[0 1 1 1-e 1-e 0+e],c3);plot([0 1 1 0 0],[0 0 1 1 0]);
  Output : Outport  InitialOutput=0
      mask Display: e = 0.06;c1 = [120 230 180]/255;c2 = ([120 230 180]+0)/(256+128);c3 = ([120 230 180]+128)/(256+128);patch([0 1 1 0],[0 0 1 1],c1);patch([0 1 1 1-e 1-e 0+e],[0 0 1 1-e 0+e 0+e],c2);patch([0 0 1 1-e 0+e 0+e],[0 1 1 1-e 1-e 0+e],c3);plot([0 1 1 0 0],[0 0 1 1 0]);
  wires:
  Layer 6/1("a{6}") -> Process Output 1/1(a)
  [feedback5] -> Layer 6/6("a{5} ")
  Layer 5/1("a{5}") -> [feedback5]
  [feedback4] -> Layer 6/5("a{4} "), Layer 5/5("a{4} ")
  Layer 4/1("a{4}") -> [feedback4]
  [feedback3] -> Layer 6/4("a{3} "), Layer 5/4("a{3} "), Layer 4/4("a{3} ")
  Layer 3/1("a{3}") -> [feedback3]
  [feedback2] -> Layer 6/3("a{2} "), Layer 5/3("a{2} "), Layer 4/3("a{2} "), Layer 3/3("a{2} ")
  Layer 2/1("a{2}") -> [feedback2]
  [feedback1] -> Layer 6/2("a{1} "), Layer 5/2("a{1} "), Layer 4/2("a{1} "), Layer 3/2("a{1} "), Layer 2/2("a{1} ")
  Layer 1/1("a{1}") -> [feedback1]
  ? -> Layer 6/1("p{1}"), Layer 5/1("p{1}"), Layer 4/1("p{1}"), Layer 3/1("p{1}"), Layer 2/1("p{1}"), Layer 1/1("p{1}")
  Process Output 1/1(y) -> Output/1
  Input/1 -> ?

== system My_Model/Subsystem1/Custom Neural Network1 ==
  Input : Inport  PortDimensions=2
      mask Display: e = 0.06;c1 = [120 230 180]/255;c2 = ([120 230 180]+0)/(256+128);c3 = ([120 230 180]+128)/(256+128);patch([0 1 1 0],[0 0 1 1],c1);patch([0 1 1 1-e 1-e 0+e],[0 0 1 1-e 0+e 0+e],c2);patch([0 0 1 1-e 0+e 0+e],[0 1 1 1-e 1-e 0+e],c3);plot([0 1 1 0 0],[0 0 1 1 0]);
  Layer 1 : Subsystem
      mask Display: e = 0.06;c1 = [120 150 230]/255;c2 = ([120 150 230]+0)/383;c3 = ([120 150 230]+128)/383;patch([0 1 1 0],[0 0 1 1],c1);patch([0 1 1 1-e 1-e 0+e],[0 0 1 1-e 0+e 0+e],c2);patch([0 0 1 1-e 0+e 0+e],[0 1 1 1-e 1-e 0+e],c3);plot([0 1 1 0 0],[0 0 1 1 0]);
  Layer 2 : Subsystem
      mask Display: e = 0.06;c1 = [120 150 230]/255;c2 = ([120 150 230]+0)/383;c3 = ([120 150 230]+128)/383;patch([0 1 1 0],[0 0 1 1],c1);patch([0 1 1 1-e 1-e 0+e],[0 0 1 1-e 0+e 0+e],c2);patch([0 0 1 1-e 0+e 0+e],[0 1 1 1-e 1-e 0+e],c3);plot([0 1 1 0 0],[0 0 1 1 0]);
  Layer 3 : Subsystem
      mask Display: e = 0.06;c1 = [120 150 230]/255;c2 = ([120 150 230]+0)/383;c3 = ([120 150 230]+128)/383;patch([0 1 1 0],[0 0 1 1],c1);patch([0 1 1 1-e 1-e 0+e],[0 0 1 1-e 0+e 0+e],c2);patch([0 0 1 1-e 0+e 0+e],[0 1 1 1-e 1-e 0+e],c3);plot([0 1 1 0 0],[0 0 1 1 0]);
  Layer 4 : Subsystem
      mask Display: e = 0.06;c1 = [120 150 230]/255;c2 = ([120 150 230]+0)/383;c3 = ([120 150 230]+128)/383;patch([0 1 1 0],[0 0 1 1],c1);patch([0 1 1 1-e 1-e 0+e],[0 0 1 1-e 0+e 0+e],c2);patch([0 0 1 1-e 0+e 0+e],[0 1 1 1-e 1-e 0+e],c3);plot([0 1 1 0 0],[0 0 1 1 0]);
  Layer 5 : Subsystem
      mask Display: e = 0.06;c1 = [120 150 230]/255;c2 = ([120 150 230]+0)/383;c3 = ([120 150 230]+128)/383;patch([0 1 1 0],[0 0 1 1],c1);patch([0 1 1 1-e 1-e 0+e],[0 0 1 1-e 0+e 0+e],c2);patch([0 0 1 1-e 0+e 0+e],[0 1 1 1-e 1-e 0+e],c3);plot([0 1 1 0 0],[0 0 1 1 0]);
  Layer 6 : Subsystem
      mask Display: e = 0.06;c1 = [120 150 230]/255;c2 = ([120 150 230]+0)/383;c3 = ([120 150 230]+128)/383;patch([0 1 1 0],[0 0 1 1],c1);patch([0 1 1 1-e 1-e 0+e],[0 0 1 1-e 0+e 0+e],c2);patch([0 0 1 1-e 0+e 0+e],[0 1 1 1-e 1-e 0+e],c3);plot([0 1 1 0 0],[0 0 1 1 0]);
  Process Output 1 : Subsystem
      mask Display: e = 0.06;c1 = [120 150 230]/255;c2 = ([120 150 230]+0)/383;c3 = ([120 150 230]+128)/383;patch([0 1 1 0],[0 0 1 1],c1);patch([0 1 1 1-e 1-e 0+e],[0 0 1 1-e 0+e 0+e],c2);patch([0 0 1 1-e 0+e 0+e],[0 1 1 1-e 1-e 0+e],c3);plot([0 1 1 0 0],[0 0 1 1 0]);
  Output : Outport  InitialOutput=0
      mask Display: e = 0.06;c1 = [120 230 180]/255;c2 = ([120 230 180]+0)/(256+128);c3 = ([120 230 180]+128)/(256+128);patch([0 1 1 0],[0 0 1 1],c1);patch([0 1 1 1-e 1-e 0+e],[0 0 1 1-e 0+e 0+e],c2);patch([0 0 1 1-e 0+e 0+e],[0 1 1 1-e 1-e 0+e],c3);plot([0 1 1 0 0],[0 0 1 1 0]);
  wires:
  Layer 6/1("a{6}") -> Process Output 1/1(a)
  [feedback5] -> Layer 6/6("a{5} ")
  Layer 5/1("a{5}") -> [feedback5]
  [feedback4] -> Layer 6/5("a{4} "), Layer 5/5("a{4} ")
  Layer 4/1("a{4}") -> [feedback4]
  [feedback3] -> Layer 6/4("a{3} "), Layer 5/4("a{3} "), Layer 4/4("a{3} ")
  Layer 3/1("a{3}") -> [feedback3]
  [feedback2] -> Layer 6/3("a{2} "), Layer 5/3("a{2} "), Layer 4/3("a{2} "), Layer 3/3("a{2} ")
  Layer 2/1("a{2}") -> [feedback2]
  [feedback1] -> Layer 6/2("a{1} "), Layer 5/2("a{1} "), Layer 4/2("a{1} "), Layer 3/2("a{1} "), Layer 2/2("a{1} ")
  Layer 1/1("a{1}") -> [feedback1]
  ? -> Layer 6/1("p{1}"), Layer 5/1("p{1}"), Layer 4/1("p{1}"), Layer 3/1("p{1}"), Layer 2/1("p{1}"), Layer 1/1("p{1}")
  Process Output 1/1(y) -> Output/1
  Input/1 -> ?

== system My_Model/Subsystem2/Custom Neural Network1 ==
  Input : Inport  PortDimensions=2
      mask Display: e = 0.06;c1 = [120 230 180]/255;c2 = ([120 230 180]+0)/(256+128);c3 = ([120 230 180]+128)/(256+128);patch([0 1 1 0],[0 0 1 1],c1);patch([0 1 1 1-e 1-e 0+e],[0 0 1 1-e 0+e 0+e],c2);patch([0 0 1 1-e 0+e 0+e],[0 1 1 1-e 1-e 0+e],c3);plot([0 1 1 0 0],[0 0 1 1 0]);
  Layer 1 : Subsystem
      mask Display: e = 0.06;c1 = [120 150 230]/255;c2 = ([120 150 230]+0)/383;c3 = ([120 150 230]+128)/383;patch([0 1 1 0],[0 0 1 1],c1);patch([0 1 1 1-e 1-e 0+e],[0 0 1 1-e 0+e 0+e],c2);patch([0 0 1 1-e 0+e 0+e],[0 1 1 1-e 1-e 0+e],c3);plot([0 1 1 0 0],[0 0 1 1 0]);
  Layer 2 : Subsystem
      mask Display: e = 0.06;c1 = [120 150 230]/255;c2 = ([120 150 230]+0)/383;c3 = ([120 150 230]+128)/383;patch([0 1 1 0],[0 0 1 1],c1);patch([0 1 1 1-e 1-e 0+e],[0 0 1 1-e 0+e 0+e],c2);patch([0 0 1 1-e 0+e 0+e],[0 1 1 1-e 1-e 0+e],c3);plot([0 1 1 0 0],[0 0 1 1 0]);
  Layer 3 : Subsystem
      mask Display: e = 0.06;c1 = [120 150 230]/255;c2 = ([120 150 230]+0)/383;c3 = ([120 150 230]+128)/383;patch([0 1 1 0],[0 0 1 1],c1);patch([0 1 1 1-e 1-e 0+e],[0 0 1 1-e 0+e 0+e],c2);patch([0 0 1 1-e 0+e 0+e],[0 1 1 1-e 1-e 0+e],c3);plot([0 1 1 0 0],[0 0 1 1 0]);
  Layer 4 : Subsystem
      mask Display: e = 0.06;c1 = [120 150 230]/255;c2 = ([120 150 230]+0)/383;c3 = ([120 150 230]+128)/383;patch([0 1 1 0],[0 0 1 1],c1);patch([0 1 1 1-e 1-e 0+e],[0 0 1 1-e 0+e 0+e],c2);patch([0 0 1 1-e 0+e 0+e],[0 1 1 1-e 1-e 0+e],c3);plot([0 1 1 0 0],[0 0 1 1 0]);
  Layer 5 : Subsystem
      mask Display: e = 0.06;c1 = [120 150 230]/255;c2 = ([120 150 230]+0)/383;c3 = ([120 150 230]+128)/383;patch([0 1 1 0],[0 0 1 1],c1);patch([0 1 1 1-e 1-e 0+e],[0 0 1 1-e 0+e 0+e],c2);patch([0 0 1 1-e 0+e 0+e],[0 1 1 1-e 1-e 0+e],c3);plot([0 1 1 0 0],[0 0 1 1 0]);
  Layer 6 : Subsystem
      mask Display: e = 0.06;c1 = [120 150 230]/255;c2 = ([120 150 230]+0)/383;c3 = ([120 150 230]+128)/383;patch([0 1 1 0],[0 0 1 1],c1);patch([0 1 1 1-e 1-e 0+e],[0 0 1 1-e 0+e 0+e],c2);patch([0 0 1 1-e 0+e 0+e],[0 1 1 1-e 1-e 0+e],c3);plot([0 1 1 0 0],[0 0 1 1 0]);
  Process Output 1 : Subsystem
      mask Display: e = 0.06;c1 = [120 150 230]/255;c2 = ([120 150 230]+0)/383;c3 = ([120 150 230]+128)/383;patch([0 1 1 0],[0 0 1 1],c1);patch([0 1 1 1-e 1-e 0+e],[0 0 1 1-e 0+e 0+e],c2);patch([0 0 1 1-e 0+e 0+e],[0 1 1 1-e 1-e 0+e],c3);plot([0 1 1 0 0],[0 0 1 1 0]);
  Output : Outport  InitialOutput=0
      mask Display: e = 0.06;c1 = [120 230 180]/255;c2 = ([120 230 180]+0)/(256+128);c3 = ([120 230 180]+128)/(256+128);patch([0 1 1 0],[0 0 1 1],c1);patch([0 1 1 1-e 1-e 0+e],[0 0 1 1-e 0+e 0+e],c2);patch([0 0 1 1-e 0+e 0+e],[0 1 1 1-e 1-e 0+e],c3);plot([0 1 1 0 0],[0 0 1 1 0]);
  wires:
  Layer 6/1("a{6}") -> Process Output 1/1(a)
  [feedback5] -> Layer 6/6("a{5} ")
  Layer 5/1("a{5}") -> [feedback5]
  [feedback4] -> Layer 6/5("a{4} "), Layer 5/5("a{4} ")
  Layer 4/1("a{4}") -> [feedback4]
  [feedback3] -> Layer 6/4("a{3} "), Layer 5/4("a{3} "), Layer 4/4("a{3} ")
  Layer 3/1("a{3}") -> [feedback3]
  [feedback2] -> Layer 6/3("a{2} "), Layer 5/3("a{2} "), Layer 4/3("a{2} "), Layer 3/3("a{2} ")
  Layer 2/1("a{2}") -> [feedback2]
  [feedback1] -> Layer 6/2("a{1} "), Layer 5/2("a{1} "), Layer 4/2("a{1} "), Layer 3/2("a{1} "), Layer 2/2("a{1} ")
  Layer 1/1("a{1}") -> [feedback1]
  ? -> Layer 6/1("p{1}"), Layer 5/1("p{1}"), Layer 4/1("p{1}"), Layer 3/1("p{1}"), Layer 2/1("p{1}"), Layer 1/1("p{1}")
  Process Output 1/1(y) -> Output/1
  Input/1 -> ?
